simulink subsystem "SelfDefined_Buck_Converter"  (R2024b)
settings: Solver=VariableStepAuto  StartTime=0.0  StopTime=10.0  RelTol=1e-3
libraries: simulink x1, spsDiodeLib x1, spsIGBTLib x1
settings Model: Creator=XixiLab  LastModifiedBy=XixiLab

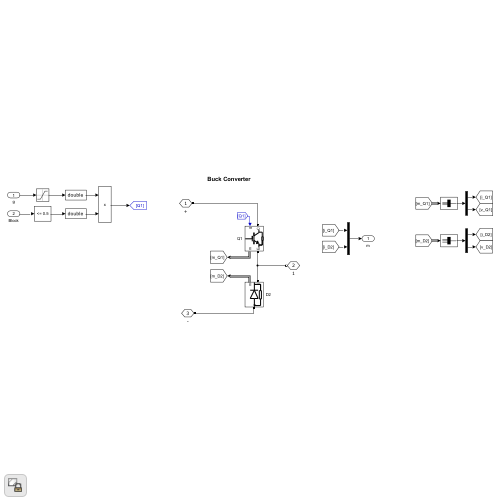
[thumbnail: Simulink's stored preview of the top-level diagram]
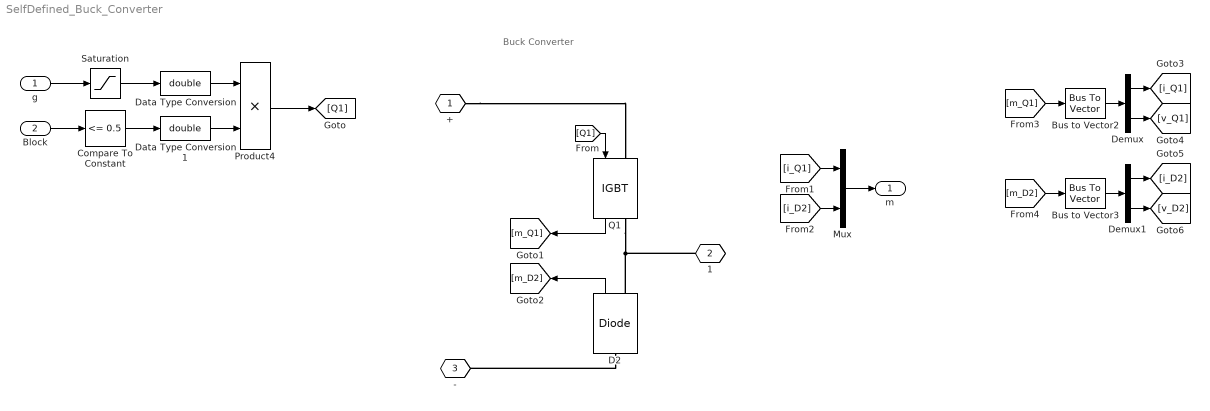
== system SelfDefined_Buck_Converter ==
  note: Buck Converter
  g : Inport  PortDimensions=1
  Block : Inport  Port=2  PortDimensions=1
  Bus to Vector2 : BusToVector
  Bus to Vector3 : BusToVector
  Compare To Constant : simulink/Logic and Bit Operations/Compare To Constant  relop=<=  const=0.5  OutDataTypeStr=boolean
  D2 : spsDiodeLib/Diode  Ron=0.001  Lon=0  Vf=0  IC=0  UseSnubber=0  Rs=1e6  Cs=inf  Measurements=on
  Data Type Conversion : DataTypeConversion  OutDataTypeStr=double  SaturateOnIntegerOverflow=off  RndMeth=Floor
  Data Type Conversion1 : DataTypeConversion  OutDataTypeStr=double  SaturateOnIntegerOverflow=off  RndMeth=Floor
  Demux : Demux  Outputs=2
  Demux1 : Demux  Outputs=2
  Mux : Mux  Inputs=2
  Product4 : Product
  Q1 : spsIGBTLib/IGBT  Ron=0.001  Lon=0  Vf=0  Tf=1e-6  Tt=2e-6  IC=0  Rs=1e5  Cs=inf  Measurements=on
  Saturation : Saturate  UpperLimit=1  LowerLimit=0
  + : PMIOPort  Tag=PMCPort  Side=Right
  1 : PMIOPort  Tag=PMCPort  Port=2  Side=Left
  - : PMIOPort  Tag=PMCPort  Port=3  Side=Right
  m : Outport
  wires:
  Compare To Constant/1 -> Data Type Conversion1/1
  Block/1 -> Compare To Constant/1
  g/1 -> Saturation/1
  Data Type Conversion/1 -> Product4/1
  [Q1] -> Q1/1
  Saturation/1 -> Data Type Conversion/1
  Product4/1 -> [Q1]
  Data Type Conversion1/1 -> Product4/2
  Q1/1 -> [m_Q1]
  D2/1 -> [m_D2]
  Mux/1 -> m/1
  [i_Q1] -> Mux/1
  [i_D2] -> Mux/2
  [m_D2] -> Bus to Vector3/1
  [m_Q1] -> Bus to Vector2/1
  Bus to Vector2/1 -> Demux/1
  Demux/1 -> [i_Q1]
  Demux/2 -> [v_Q1]
  Demux1/2 -> [v_D2]
  Bus to Vector3/1 -> Demux1/1
  Demux1/1 -> [i_D2]
  connections:
  D2/RConn1 -- Q1/RConn1 -- 1/RConn1
  +/RConn1 -- Q1/LConn1
  D2/LConn1 -- -/RConn1
